simulink library "aerolib3dofsys"  (Simulink 5.0)
undefined symbols (not defined in the file or in its folder): Iyy, mass, mass_e, mass_f
libraries: aerolibbdyn x1
settings Model: Creator=sgage  LastModifiedBy=sgage

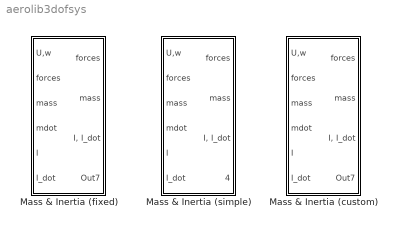
== system aerolib3dofsys ==
  Mass & Inertia (custom) : Subsystem
      mask Type: Mass & Inertia (custom)
  Mass & Inertia (fixed) : Subsystem
      mask Type: Mass & Inertia (fixed)
  Mass & Inertia (simple) : Subsystem
      mask Type: Mass & Inertia (simple)

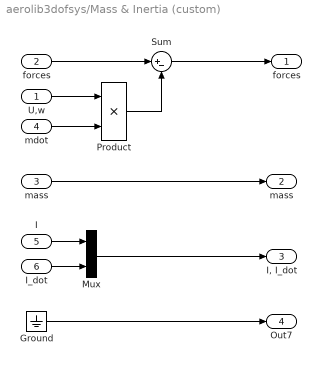
== system aerolib3dofsys/Mass & Inertia (custom) ==
  U,w : Inport
  forces : Inport  Port=2
  "mass  " : Inport  Port=3
  mdot : Inport  Port=4
  I : Inport  Port=5  ShowAdditionalParam=on  DataType=double
  I_dot : Inport  Port=6  ShowAdditionalParam=on  DataType=double
  Ground : Ground
  Mux : Mux  Inputs=2
  Product : Product  SaturateOnIntegerOverflow=on
  Sum : Sum  Inputs=|+-  SaturateOnIntegerOverflow=on
  "forces " : Outport
  "mass " : Outport  Port=2
  "I, I_dot" : Outport  Port=3
  Out7 : Outport  Port=4
  wires:
  Sum/1 -> "forces "/1
  forces/1 -> Sum/1
  U,w/1 -> Product/1
  Product/1 -> Sum/2
  I/1 -> Mux/1
  I_dot/1 -> Mux/2
  "mass  "/1 -> "mass "/1
  Mux/1 -> "I, I_dot"/1
  Ground/1 -> Out7/1
  mdot/1 -> Product/2

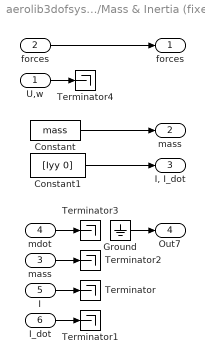
== system aerolib3dofsys/Mass & Inertia (fixed) ==
  U,w : Inport
  forces : Inport  Port=2
  "mass  " : Inport  Port=3
  mdot : Inport  Port=4
  I : Inport  Port=5  ShowAdditionalParam=on  DataType=double
  I_dot : Inport  Port=6  ShowAdditionalParam=on  DataType=double
  Constant : Constant  Value=mass  ShowAdditionalParam=on
  Constant1 : Constant  Value=[Iyy 0]  ShowAdditionalParam=on
  Ground : Ground
  Terminator{,1..4} (5 alike) : Terminator
  "forces " : Outport
  "mass " : Outport  Port=2
  "I, I_dot" : Outport  Port=3
  Out7 : Outport  Port=4
  wires:
  Constant/1 -> "mass "/1
  forces/1 -> "forces "/1
  U,w/1 -> Terminator4/1
  I/1 -> Terminator/1
  I_dot/1 -> Terminator1/1
  "mass  "/1 -> Terminator2/1
  Constant1/1 -> "I, I_dot"/1
  Ground/1 -> Out7/1
  mdot/1 -> Terminator3/1

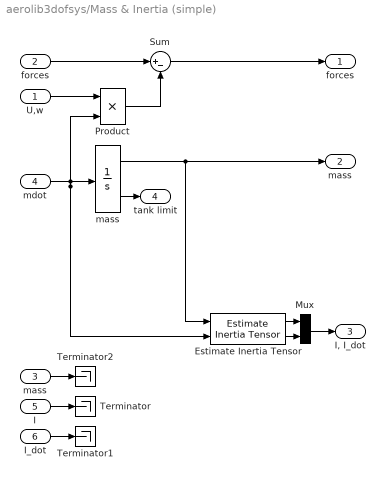
== system aerolib3dofsys/Mass & Inertia (simple) ==
  U,w : Inport
  forces : Inport  Port=2
  "mass  " : Inport  Port=3
  mdot : Inport  Port=4
  I : Inport  Port=5  ShowAdditionalParam=on  DataType=double
  I_dot : Inport  Port=6  ShowAdditionalParam=on  DataType=double
  Estimate Inertia Tensor : aerolibbdyn/Estimate Inertia Tensor  fmass=mass_f  emass=mass_e  fI=Iyy_f  eI=Iyy_e
  Mux : Mux  Inputs=2
  Product : Product  SaturateOnIntegerOverflow=on
  Sum : Sum  Inputs=|+-  SaturateOnIntegerOverflow=on
  Terminator : Terminator
  Terminator1 : Terminator
  Terminator2 : Terminator
  mass : Integrator  InitialCondition=mass  LimitOutput=on  UpperSaturationLimit=mass_f  LowerSaturationLimit=mass_e  ShowSaturationPort=on
  "forces " : Outport
  "mass " : Outport  Port=2
  "I, I_dot" : Outport  Port=3
  tank limit : Outport  Port=4
  wires:
  mass/1 -> "mass "/1, Estimate Inertia Tensor/1
  mdot/1 -> mass/1, Estimate Inertia Tensor/2, Product/2
  mass/2 -> tank limit/1
  Estimate Inertia Tensor/1 -> Mux/1
  Estimate Inertia Tensor/2 -> Mux/2
  Mux/1 -> "I, I_dot"/1
  "mass  "/1 -> Terminator2/1
  I_dot/1 -> Terminator1/1
  I/1 -> Terminator/1
  Product/1 -> Sum/2
  U,w/1 -> Product/1
  forces/1 -> Sum/1
  Sum/1 -> "forces "/1
